simulink model "lead"  (R2017a)
settings: Solver=VariableStepAuto  StartTime=0.0  StopTime=10.0  RelTol=1e-3
settings Model: Creator=Mat Haskell  LastModifiedBy=Mat Haskell

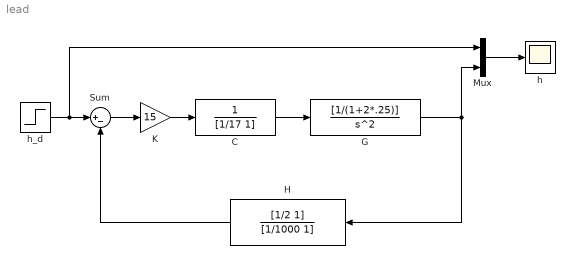
== system lead ==
  C : TransferFcn  Denominator=[1/17 1]
  G : TransferFcn  Numerator=[1/(1+2*.25)]  Denominator=[1 0 0]
  H : TransferFcn  Numerator=[1/2 1]  Denominator=[1/1000 1]
  K : Gain  Gain=15
  Mux : Mux  Inputs=2
  Sum : Sum  Inputs=|+-
  h : Scope
  h_d : Step  SampleTime=0
  wires:
  h_d/1 -> Mux/1, Sum/1
  Sum/1 -> K/1
  K/1 -> C/1
  C/1 -> G/1
  G/1 -> H/1, Mux/2
  H/1 -> Sum/2
  Mux/1 -> h/1
